simulink model "dois"  (R2022b)
settings: Solver=VariableStepAuto  StartTime=0.0  StopTime=10.0  RelTol=1e-3
settings Model: Creator=Admin  LastModifiedBy=Admin

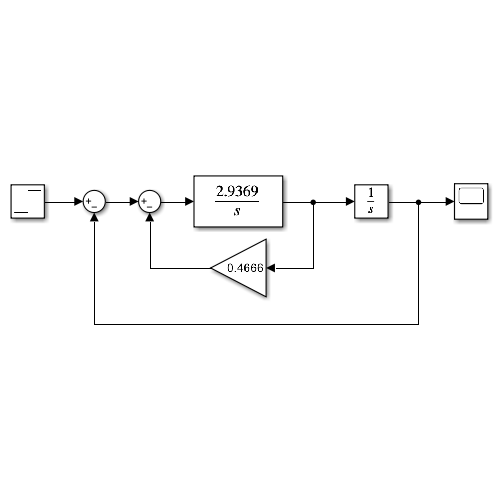
[thumbnail: Simulink's stored preview of the top-level diagram]
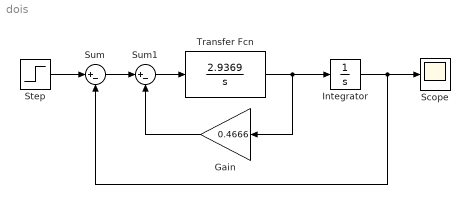
== system dois ==
  Gain : Gain  Gain=0.4666
  Integrator : Integrator
  Scope : Scope
  Step : Step  SampleTime=0
  Sum : Sum  Inputs=|+-
  Sum1 : Sum  Inputs=|+-
  Transfer Fcn : TransferFcn  Numerator=[2.9369]  Denominator=[1 0]
  wires:
  Step/1 -> Sum/1
  Sum/1 -> Sum1/1
  Sum1/1 -> Transfer Fcn/1
  Transfer Fcn/1 -> Gain/1, Integrator/1
  Gain/1 -> Sum1/2
  Integrator/1 -> Sum/2, Scope/1
